simulink model "ScriptDemo"  (R2022b)
settings: configuration reference "TmVcThermal_Configuration_sub" (kept outside this file)
undefined symbols (not defined in the file): aaaa, bbbb, cTmComprCtrl_D_u8HvacFlowTable_db, cTmComprCtrl_D_u8HvacFlowTable_sw, cTmComprCtrl_n_i16ChillCmpIMax, cTmComprCtrl_n_i16ChillCmpIMin, cTmComprCtrl_n_i16ChillCmpIMin666, cTmComprCtrl_n_i16ChillCmpPMax, cTmComprCtrl_n_i16ChillCmpPMin, cTmComprCtrl_n_i16CmpChillCoolRpmKiMax, cTmComprCtrl_n_i16CmpChillCoolRpmKiMin, cTmComprCtrl_n_i16CmpChillCoolRpmKpMax, cTmComprCtrl_n_i16CmpChillCoolRpmKpMin, cTmComprCtrl_n_i16CmpCoolRpmKiMax, cTmComprCtrl_n_i16CmpCoolRpmKiMin, cTmComprCtrl_n_i16CmpCoolRpmKpMax, cTmComprCtrl_n_i16CmpCoolRpmKpMin, cTmComprCtrl_n_i16SM4CmpHeatKiMax, cTmComprCtrl_n_i16SM4CmpHeatKiMin, cTmComprCtrl_n_i16SM4CmpHeatKpMax, cTmComprCtrl_n_i16SM4CmpHeatKpMin, cTmComprCtrl_n_i16SM5CmpHeatKiMax, cTmComprCtrl_n_i16SM5CmpHeatKiMin, cTmComprCtrl_n_i16SM5CmpHeatKpMax, cTmComprCtrl_n_i16SM5CmpHeatKpMin, cTmComprCtrl_n_i16SM6CmpHeatKiMax, cTmComprCtrl_n_i16SM6CmpHeatKiMin, cTmComprCtrl_n_i16SM6CmpHeatKpMax, cTmComprCtrl_n_i16SM6CmpHeatKpMin, cTmComprCtrl_n_u16CmpMaxSpdFanFltLimt, cTmComprCtrl_n_u16CmpMaxSpdLoSidePFltLimt, cTmComprCtrl_n_u16CmpMaxSpdSensorFltLimt, cTmComprCtrl_n_u16CompMinRpm, cTmComprCtrl_n_u16CompRpmIncThres, cTmComprCtrl_t_u16BattCooltFFPeriod, cTmComprCtrl_t_u16BattCooltPIPeriod, cTmComprCtrl_t_u16CmpCoolFFPeriod, cTmComprCtrl_t_u16CmpCoolPIPeriod, cTmComprCtrl_t_u16CoolCmpChillFFPeriod, cTmComprCtrl_t_u16CoolCmpChillPIPeriod, cTmComprCtrl_t_u16SM4CmpHeatFFPeriod, cTmComprCtrl_t_u16SM4CmpHeatPIPeriod, cTmComprCtrl_t_u16SM5CmpHeatFFPeriod, cTmComprCtrl_t_u16SM5CmpHeatPIPeriod, cTmComprCtrl_t_u16SM6CmpHeatFFPeriod, cTmComprCtrl_t_u16SM6CmpHeatPIPeriod, cTmComprCtrl_Te_EvapClearInteg, cTmComprCtrl_Te_i16HpReqTempSaturoffset, cTmComprCtrl_Te_i16SatLpReplaceDiff, cTmComprCtrl_Te_i16SM3BatDiffStartEvapDecOffset, cTmComprCtrl_Te_i16SM3EvapLo, cTmComprCtrl_Te_i16SM3TBatDiffEntEvapDecOffset, cTmComprCtrl_Te_i16SM3TBatDiffEntEvapDecOffsetQuit, cTmComprCtrl_Te_s32ErrCmpChillPIContinueCoolH, cTmComprCtrl_Te_s32ErrCmpChillPIContinueCoolL, cTmComprCtrl_Te_s32ErrCmpPIContinueChillH, cTmComprCtrl_Te_s32ErrCmpPIContinueChillL, cTmComprCtrl_Te_s32ErrCmpPIContinueCoolH, cTmComprCtrl_Te_s32ErrCmpPIContinueCoolL, cTmComprCtrl_Te_s32ErrCmpPIContinueHeatH ... (+398)
libraries: simulink x782, PCMULib x640, simulink_need_slupdate x4
(part 31 of 41)

== system ScriptDemo/Create/createMerge/After/SM2SM22/SM2_Kp/Osa/Subsystem1 ==
  In1 : Inport  OutDataTypeStr=int16
  Abs : Abs  OutDataTypeStr=single  SaturateOnIntegerOverflow=off
  Add6 : Sum  Inputs=+-  OutDataTypeStr=int16
  Compare To Constant : simulink/Logic and Bit Operations/Compare To Constant  relop=>=  const=0  OutDataTypeStr=boolean
  Compare To Constant1 : simulink/Logic and Bit Operations/Compare To Constant  relop=<=  const=10  OutDataTypeStr=boolean
  Constant6 : Constant  Value=0  OutDataTypeStr=uint16
  Constant7 : Constant  Value=10  OutDataTypeStr=uint16
  Logical Operator : Logic  AllPortsSameDT=off  OutDataTypeStr=boolean
  Switch : Switch  Criteria=u2 ~= 0  SaturateOnIntegerOverflow=off  InputSameDT=off
  Out1 : Outport
  wires:
  Add6/1 -> Switch/1
  Logical Operator/1 -> Switch/2
  Constant6/1 -> Switch/3
  Abs/1 -> Add6/2, Compare To Constant/1, Compare To Constant1/1
  Constant7/1 -> Add6/1
  Switch/1 -> Out1/1
  Compare To Constant1/1 -> Logical Operator/2
  Compare To Constant/1 -> Logical Operator/1
  In1/1 -> Abs/1

== system ScriptDemo/Create/createMerge/After/SM2SM22/SM2_Kp/Osa/Subsystem2 ==
  In1 : Inport  OutDataTypeStr=int16
  Abs : Abs  OutDataTypeStr=uint16  SaturateOnIntegerOverflow=off
  Add6 : Sum  Inputs=+-  OutDataTypeStr=int16
  Compare To Constant : simulink/Logic and Bit Operations/Compare To Constant  relop=>=  const=0  OutDataTypeStr=boolean
  Compare To Constant1 : simulink/Logic and Bit Operations/Compare To Constant  relop=<=  const=10  OutDataTypeStr=boolean
  Constant6 : Constant  Value=0  OutDataTypeStr=uint16
  Constant7 : Constant  Value=10  OutDataTypeStr=uint16
  Logical Operator : Logic  AllPortsSameDT=off  OutDataTypeStr=boolean
  Switch : Switch  Criteria=u2 ~= 0  SaturateOnIntegerOverflow=off  InputSameDT=off
  Out1 : Outport
  wires:
  Add6/1 -> Switch/1
  Logical Operator/1 -> Switch/2
  Constant6/1 -> Switch/3
  Abs/1 -> Add6/2, Compare To Constant/1, Compare To Constant1/1
  Constant7/1 -> Add6/1
  Switch/1 -> Out1/1
  Compare To Constant1/1 -> Logical Operator/2
  Compare To Constant/1 -> Logical Operator/1
  In1/1 -> Abs/1

== system ScriptDemo/Create/createMerge/After/SM2SM22/SM2_Kp/Osa/Subsystem3 ==
  In1 : Inport  OutDataTypeStr=int16
  Abs : Abs  OutDataTypeStr=uint16  SaturateOnIntegerOverflow=off
  Add6 : Sum  Inputs=+-  OutDataTypeStr=int16
  Compare To Constant : simulink/Logic and Bit Operations/Compare To Constant  relop=>=  const=0  OutDataTypeStr=boolean
  Compare To Constant1 : simulink/Logic and Bit Operations/Compare To Constant  relop=<=  const=10  OutDataTypeStr=boolean
  Constant6 : Constant  Value=0  OutDataTypeStr=uint16
  Constant7 : Constant  Value=10  OutDataTypeStr=uint16
  Logical Operator : Logic  AllPortsSameDT=off  OutDataTypeStr=boolean
  Switch : Switch  Criteria=u2 ~= 0  SaturateOnIntegerOverflow=off  InputSameDT=off
  Out1 : Outport
  wires:
  Add6/1 -> Switch/1
  Logical Operator/1 -> Switch/2
  Constant6/1 -> Switch/3
  Abs/1 -> Add6/2, Compare To Constant/1, Compare To Constant1/1
  Constant7/1 -> Add6/1
  Switch/1 -> Out1/1
  Compare To Constant1/1 -> Logical Operator/2
  Compare To Constant/1 -> Logical Operator/1
  In1/1 -> Abs/1

== system ScriptDemo/Create/createMerge/After/SM2SM22/SM2_Kp/Osa/Subsystem4 ==
  In1 : Inport  OutDataTypeStr=int16
  Abs : Abs  OutDataTypeStr=uint16  SaturateOnIntegerOverflow=off
  Add6 : Sum  Inputs=+-  OutDataTypeStr=int16
  Compare To Constant : simulink/Logic and Bit Operations/Compare To Constant  relop=>=  const=0  OutDataTypeStr=boolean
  Compare To Constant1 : simulink/Logic and Bit Operations/Compare To Constant  relop=<=  const=10  OutDataTypeStr=boolean
  Constant6 : Constant  Value=0  OutDataTypeStr=uint16
  Constant7 : Constant  Value=10  OutDataTypeStr=uint16
  Logical Operator : Logic  AllPortsSameDT=off  OutDataTypeStr=boolean
  Switch : Switch  Criteria=u2 ~= 0  SaturateOnIntegerOverflow=off  InputSameDT=off
  Out1 : Outport
  wires:
  Add6/1 -> Switch/1
  Logical Operator/1 -> Switch/2
  Constant6/1 -> Switch/3
  Abs/1 -> Add6/2, Compare To Constant/1, Compare To Constant1/1
  Constant7/1 -> Add6/1
  Switch/1 -> Out1/1
  Compare To Constant1/1 -> Logical Operator/2
  Compare To Constant/1 -> Logical Operator/1
  In1/1 -> Abs/1

== system ScriptDemo/Create/createMerge/After/SM2SM22/SM2_Kp/Osa/Subsystem5 ==
  In1 : Inport  OutDataTypeStr=int16
  Abs : Abs  OutDataTypeStr=uint16  SaturateOnIntegerOverflow=off
  Add6 : Sum  Inputs=+-  OutDataTypeStr=int16
  Compare To Constant : simulink/Logic and Bit Operations/Compare To Constant  relop=>=  const=0  OutDataTypeStr=boolean
  Compare To Constant1 : simulink/Logic and Bit Operations/Compare To Constant  relop=<=  const=10  OutDataTypeStr=boolean
  Constant6 : Constant  Value=0  OutDataTypeStr=uint16
  Constant7 : Constant  Value=10  OutDataTypeStr=uint16
  Logical Operator : Logic  AllPortsSameDT=off  OutDataTypeStr=boolean
  Switch : Switch  Criteria=u2 ~= 0  SaturateOnIntegerOverflow=off  InputSameDT=off
  Out1 : Outport
  wires:
  Add6/1 -> Switch/1
  Logical Operator/1 -> Switch/2
  Constant6/1 -> Switch/3
  Abs/1 -> Add6/2, Compare To Constant/1, Compare To Constant1/1
  Constant7/1 -> Add6/1
  Switch/1 -> Out1/1
  Compare To Constant1/1 -> Logical Operator/2
  Compare To Constant/1 -> Logical Operator/1
  In1/1 -> Abs/1

== system ScriptDemo/Create/createMerge/After/SM2SM22/SM2_Kp/Osa/XCP ==
  md_u8Blw : Inport
  Constant1 : Constant  Value=BlwHeatLevel_db
      settings: AttributesFormatString=%<Value>
  Constant28 : Constant  Value=BlwHeatLevel_sw
      settings: AttributesFormatString=%<Value>
  Switch : Switch  Criteria=u2 ~= 0  SaturateOnIntegerOverflow=off  InputSameDT=off
  Out1 : Outport
  wires:
  md_u8Blw/1 -> Switch/3
  Switch/1 -> Out1/1
  Constant28/1 -> Switch/2
  Constant1/1 -> Switch/1

== system ScriptDemo/Create/createMerge/After/SM2SM22/SM2_Kp/Rec/Subsystem1 ==
  In1 : Inport  OutDataTypeStr=int16
  Abs : Abs  OutDataTypeStr=single  SaturateOnIntegerOverflow=off
  Add6 : Sum  Inputs=+-  OutDataTypeStr=int16
  Compare To Constant : simulink/Logic and Bit Operations/Compare To Constant  relop=>=  const=0  OutDataTypeStr=boolean
  Compare To Constant1 : simulink/Logic and Bit Operations/Compare To Constant  relop=<=  const=10  OutDataTypeStr=boolean
  Constant6 : Constant  Value=0  OutDataTypeStr=uint16
  Constant7 : Constant  Value=10  OutDataTypeStr=uint16
  Logical Operator : Logic  AllPortsSameDT=off  OutDataTypeStr=boolean
  Switch : Switch  Criteria=u2 ~= 0  SaturateOnIntegerOverflow=off  InputSameDT=off
  Out1 : Outport
  wires:
  Add6/1 -> Switch/1
  Logical Operator/1 -> Switch/2
  Constant6/1 -> Switch/3
  Abs/1 -> Add6/2, Compare To Constant/1, Compare To Constant1/1
  Constant7/1 -> Add6/1
  Switch/1 -> Out1/1
  Compare To Constant1/1 -> Logical Operator/2
  Compare To Constant/1 -> Logical Operator/1
  In1/1 -> Abs/1

== system ScriptDemo/Create/createMerge/After/SM2SM22/SM2_Kp/Rec/Subsystem2 ==
  In1 : Inport  OutDataTypeStr=int16
  Abs : Abs  OutDataTypeStr=uint16  SaturateOnIntegerOverflow=off
  Add6 : Sum  Inputs=+-  OutDataTypeStr=int16
  Compare To Constant : simulink/Logic and Bit Operations/Compare To Constant  relop=>=  const=0  OutDataTypeStr=boolean
  Compare To Constant1 : simulink/Logic and Bit Operations/Compare To Constant  relop=<=  const=10  OutDataTypeStr=boolean
  Constant6 : Constant  Value=0  OutDataTypeStr=uint16
  Constant7 : Constant  Value=10  OutDataTypeStr=uint16
  Logical Operator : Logic  AllPortsSameDT=off  OutDataTypeStr=boolean
  Switch : Switch  Criteria=u2 ~= 0  SaturateOnIntegerOverflow=off  InputSameDT=off
  Out1 : Outport
  wires:
  Add6/1 -> Switch/1
  Logical Operator/1 -> Switch/2
  Constant6/1 -> Switch/3
  Abs/1 -> Add6/2, Compare To Constant/1, Compare To Constant1/1
  Constant7/1 -> Add6/1
  Switch/1 -> Out1/1
  Compare To Constant1/1 -> Logical Operator/2
  Compare To Constant/1 -> Logical Operator/1
  In1/1 -> Abs/1

== system ScriptDemo/Create/createMerge/After/SM2SM22/SM2_Kp/Rec/Subsystem3 ==
  In1 : Inport  OutDataTypeStr=int16
  Abs : Abs  OutDataTypeStr=uint16  SaturateOnIntegerOverflow=off
  Add6 : Sum  Inputs=+-  OutDataTypeStr=int16
  Compare To Constant : simulink/Logic and Bit Operations/Compare To Constant  relop=>=  const=0  OutDataTypeStr=boolean
  Compare To Constant1 : simulink/Logic and Bit Operations/Compare To Constant  relop=<=  const=10  OutDataTypeStr=boolean
  Constant6 : Constant  Value=0  OutDataTypeStr=uint16
  Constant7 : Constant  Value=10  OutDataTypeStr=uint16
  Logical Operator : Logic  AllPortsSameDT=off  OutDataTypeStr=boolean
  Switch : Switch  Criteria=u2 ~= 0  SaturateOnIntegerOverflow=off  InputSameDT=off
  Out1 : Outport
  wires:
  Add6/1 -> Switch/1
  Logical Operator/1 -> Switch/2
  Constant6/1 -> Switch/3
  Abs/1 -> Add6/2, Compare To Constant/1, Compare To Constant1/1
  Constant7/1 -> Add6/1
  Switch/1 -> Out1/1
  Compare To Constant1/1 -> Logical Operator/2
  Compare To Constant/1 -> Logical Operator/1
  In1/1 -> Abs/1

== system ScriptDemo/Create/createMerge/After/SM2SM22/SM2_Kp/Rec/Subsystem4 ==
  In1 : Inport  OutDataTypeStr=int16
  Abs : Abs  OutDataTypeStr=uint16  SaturateOnIntegerOverflow=off
  Add6 : Sum  Inputs=+-  OutDataTypeStr=int16
  Compare To Constant : simulink/Logic and Bit Operations/Compare To Constant  relop=>=  const=0  OutDataTypeStr=boolean
  Compare To Constant1 : simulink/Logic and Bit Operations/Compare To Constant  relop=<=  const=10  OutDataTypeStr=boolean
  Constant6 : Constant  Value=0  OutDataTypeStr=uint16
  Constant7 : Constant  Value=10  OutDataTypeStr=uint16
  Logical Operator : Logic  AllPortsSameDT=off  OutDataTypeStr=boolean
  Switch : Switch  Criteria=u2 ~= 0  SaturateOnIntegerOverflow=off  InputSameDT=off
  Out1 : Outport
  wires:
  Add6/1 -> Switch/1
  Logical Operator/1 -> Switch/2
  Constant6/1 -> Switch/3
  Abs/1 -> Add6/2, Compare To Constant/1, Compare To Constant1/1
  Constant7/1 -> Add6/1
  Switch/1 -> Out1/1
  Compare To Constant1/1 -> Logical Operator/2
  Compare To Constant/1 -> Logical Operator/1
  In1/1 -> Abs/1

== system ScriptDemo/Create/createMerge/After/SM2SM22/SM2_Kp/Rec/Subsystem5 ==
  In1 : Inport  OutDataTypeStr=int16
  Abs : Abs  OutDataTypeStr=uint16  SaturateOnIntegerOverflow=off
  Add6 : Sum  Inputs=+-  OutDataTypeStr=int16
  Compare To Constant : simulink/Logic and Bit Operations/Compare To Constant  relop=>=  const=0  OutDataTypeStr=boolean
  Compare To Constant1 : simulink/Logic and Bit Operations/Compare To Constant  relop=<=  const=10  OutDataTypeStr=boolean
  Constant6 : Constant  Value=0  OutDataTypeStr=uint16
  Constant7 : Constant  Value=10  OutDataTypeStr=uint16
  Logical Operator : Logic  AllPortsSameDT=off  OutDataTypeStr=boolean
  Switch : Switch  Criteria=u2 ~= 0  SaturateOnIntegerOverflow=off  InputSameDT=off
  Out1 : Outport
  wires:
  Add6/1 -> Switch/1
  Logical Operator/1 -> Switch/2
  Constant6/1 -> Switch/3
  Abs/1 -> Add6/2, Compare To Constant/1, Compare To Constant1/1
  Constant7/1 -> Add6/1
  Switch/1 -> Out1/1
  Compare To Constant1/1 -> Logical Operator/2
  Compare To Constant/1 -> Logical Operator/1
  In1/1 -> Abs/1

== system ScriptDemo/Create/createMerge/After/SM2SM22/SM2_Kp/Rec/XCP ==
  md_u8Blw : Inport
  Constant1 : Constant  Value=BlwHeatLevel_db
      settings: AttributesFormatString=%<Value>
  Constant28 : Constant  Value=BlwHeatLevel_sw
      settings: AttributesFormatString=%<Value>
  Switch : Switch  Criteria=u2 ~= 0  SaturateOnIntegerOverflow=off  InputSameDT=off
  Out1 : Outport
  wires:
  md_u8Blw/1 -> Switch/3
  Switch/1 -> Out1/1
  Constant28/1 -> Switch/2
  Constant1/1 -> Switch/1

== system ScriptDemo/Create/createMerge/After/SM3SM23/ID26262_SM3FF/SM1FFEnable/BevvFFPeriod ==
  Counter_Reset : Inport
  Add : Sum
  Add1 : Sum  Inputs=+-
  Constant : Constant  Value=CounterLim
  Constant1 : Constant  Value=cTmSwArch_t_s32SampleTime
      settings: AttributesFormatString=%<Value>
  Constant2 : Constant  Value=0  OutDataTypeStr=single
  Constant50 : Constant  Value=cTmSwArch_t_s32SampleTime
      settings: AttributesFormatString=%<Value>
  Logical Operator : Logic  Operator=OR  AllPortsSameDT=off  OutDataTypeStr=boolean
  Relational Operator : RelationalOperator  OutDataTypeStr=boolean  RndMeth=Simplest  InputSameDT=off
  Switch : Switch  Criteria=u2 ~= 0  SaturateOnIntegerOverflow=off  InputSameDT=off
  Switch1 : Switch  Criteria=u2 ~= 0  SaturateOnIntegerOverflow=off  InputSameDT=off
  Unit Delay : UnitDelay  SampleTime=-1  HasFrameUpgradeWarning=on
  Unit Delay1 : UnitDelay  SampleTime=-1  HasFrameUpgradeWarning=on
  Counter_Trig : Outport
  wires:
  Relational Operator/1 -> Unit Delay1/1, Counter_Trig/1
  [CounterLim] -> Relational Operator/2
  Add/1 -> Unit Delay/1, Relational Operator/1
  Unit Delay/1 -> Switch/3
  Switch/1 -> Add/2
  Constant1/1 -> Add/1
  Logical Operator/1 -> Switch/2
  Counter_Reset/1 -> Switch1/2, Logical Operator/1
  Unit Delay1/1 -> Logical Operator/2
  Constant2/1 -> Switch1/3
  Switch1/1 -> Switch/1
  Add1/1 -> Switch1/1
  Constant50/1 -> Add1/2
  Constant/1 -> [CounterLim]
  [CounterLim] -> Add1/1

== system ScriptDemo/Create/createMerge/After/SM3SM23/ID26262_SM3FF/SM2FFEnable/PeriodTrig ==
  Counter_Reset : Inport
  Add : Sum
  Add1 : Sum  Inputs=+-
  Constant : Constant  Value=CounterLim
  Constant1 : Constant  Value=cTmSwArch_t_s32SampleTime
      settings: AttributesFormatString=%<Value>
  Constant2 : Constant  Value=0  OutDataTypeStr=single
  Constant50 : Constant  Value=cTmSwArch_t_s32SampleTime
      settings: AttributesFormatString=%<Value>
  Logical Operator : Logic  Operator=OR  AllPortsSameDT=off  OutDataTypeStr=boolean
  Relational Operator : RelationalOperator  OutDataTypeStr=boolean  RndMeth=Simplest  InputSameDT=off
  Switch : Switch  Criteria=u2 ~= 0  SaturateOnIntegerOverflow=off  InputSameDT=off
  Switch1 : Switch  Criteria=u2 ~= 0  SaturateOnIntegerOverflow=off  InputSameDT=off
  Unit Delay : UnitDelay  SampleTime=-1  HasFrameUpgradeWarning=on
  Unit Delay1 : UnitDelay  SampleTime=-1  HasFrameUpgradeWarning=on
  Counter_Trig : Outport
  wires:
  Relational Operator/1 -> Unit Delay1/1, Counter_Trig/1
  [CounterLim] -> Relational Operator/2
  Add/1 -> Unit Delay/1, Relational Operator/1
  Unit Delay/1 -> Switch/3
  Switch/1 -> Add/2
  Constant1/1 -> Add/1
  Logical Operator/1 -> Switch/2
  Counter_Reset/1 -> Switch1/2, Logical Operator/1
  Unit Delay1/1 -> Logical Operator/2
  Constant2/1 -> Switch1/3
  Switch1/1 -> Switch/1
  Add1/1 -> Switch1/1
  Constant50/1 -> Add1/2
  Constant/1 -> [CounterLim]
  [CounterLim] -> Add1/1

== system ScriptDemo/Create/createMerge/After/SM3SM23/ID26262_SM3FF/SM3SM2FF/Flow2RpmOsa ==
  md_u8Blw : Inport
  breakpoint1 : Inport  Port=2
  breakpoint2 : Inport  Port=3
  2-D Lookup Table5 : Lookup_n-D  BreakpointsForDimension1=FFBlw1_Y  BreakpointsForDimension2=FFBlw1_X  BreakpointsForDimension1DataTypeStr=Inherit: Inherit from 'Breakpoint data'  BreakpointsForDimension2DataTypeStr=Inherit: Inherit from 'Breakpoint data'  Table=FFBlw1  TableDataTypeStr=Inherit: Inherit from 'Table data'  ExtrapMethod=Clip  InternalRulePriority=Speed  OutDataTypeStr=Inherit: Inherit from 'Table data'  RndMeth=Simplest
      settings: InputPortMap=u0,u1
  2-D Lookup Table6 : Lookup_n-D  BreakpointsForDimension1=FFBlw3_Y  BreakpointsForDimension2=FFBlw3_X  BreakpointsForDimension1DataTypeStr=Inherit: Inherit from 'Breakpoint data'  BreakpointsForDimension2DataTypeStr=Inherit: Inherit from 'Breakpoint data'  Table=FFBlw3  TableDataTypeStr=Inherit: Inherit from 'Table data'  ExtrapMethod=Clip  InternalRulePriority=Speed  OutDataTypeStr=Inherit: Inherit from 'Table data'  RndMeth=Simplest
      settings: InputPortMap=u0,u1
  2-D Lookup Table7 : Lookup_n-D  BreakpointsForDimension1=FFBlw5_Y  BreakpointsForDimension2=FFBlw5_X  BreakpointsForDimension1DataTypeStr=Inherit: Inherit from 'Breakpoint data'  BreakpointsForDimension2DataTypeStr=Inherit: Inherit from 'Breakpoint data'  Table=FFBlw5  TableDataTypeStr=Inherit: Inherit from 'Table data'  ExtrapMethod=Clip  InternalRulePriority=Speed  OutDataTypeStr=Inherit: Inherit from 'Table data'  RndMeth=Simplest
      settings: InputPortMap=u0,u1
  2-D Lookup Table8 : Lookup_n-D  BreakpointsForDimension1=FFBlw7_Y  BreakpointsForDimension2=FFBlw7_X  BreakpointsForDimension1DataTypeStr=Inherit: Inherit from 'Breakpoint data'  BreakpointsForDimension2DataTypeStr=Inherit: Inherit from 'Breakpoint data'  Table=FFBlw7  TableDataTypeStr=Inherit: Inherit from 'Table data'  ExtrapMethod=Clip  InternalRulePriority=Speed  OutDataTypeStr=Inherit: Inherit from 'Table data'  RndMeth=Simplest
      settings: InputPortMap=u0,u1
  2-D Lookup Table9 : Lookup_n-D  BreakpointsForDimension1=FFBlw9_Y  BreakpointsForDimension2=FFBlw9_X  BreakpointsForDimension1DataTypeStr=Inherit: Inherit from 'Breakpoint data'  BreakpointsForDimension2DataTypeStr=Inherit: Inherit from 'Breakpoint data'  Table=FFBlw9  TableDataTypeStr=Inherit: Inherit from 'Table data'  ExtrapMethod=Clip  InternalRulePriority=Speed  OutDataTypeStr=Inherit: Inherit from 'Table data'  RndMeth=Simplest
      settings: InputPortMap=u0,u1
  Add{2..6} (5 alike) : Sum  Inputs=+-  OutDataTypeStr=int16
  Add7 : Sum  Inputs=+++++
  Constant{,1..4} (5 alike) : Constant  Value=0.1  OutDataTypeStr=single
  Constant5 : Constant  Value=10  OutDataTypeStr=int16
  Constant6 : Constant  Value=20  OutDataTypeStr=int16
  Constant7 : Constant  Value=30  OutDataTypeStr=int16
  Constant8 : Constant  Value=40  OutDataTypeStr=int16
  Constant9 : Constant  Value=50  OutDataTypeStr=int16
  Data Type Conversion : DataTypeConversion  OutDataTypeStr=uint16  SaturateOnIntegerOverflow=off  RndMeth=Floor
  Data Type Conversion1 : DataTypeConversion  OutDataTypeStr=int16  SaturateOnIntegerOverflow=off  RndMeth=Floor
  Product{,1..9} (10 alike) : Product  OutDataTypeStr=single
  Subsystem1 : Subsystem
  Subsystem2 : Subsystem
  Subsystem3 : Subsystem
  Subsystem4 : Subsystem
  Subsystem5 : Subsystem
  XCP : Subsystem
  Flow2Rpm : Outport
  wires:
  Subsystem1/1(Out1) -> Product/2
  Product2/1 -> Product7/2
  [breakpoint2] -> 2-D Lookup Table5/2
  Product4/1 -> Product9/2
  Product9/1 -> Add7/5
  [breakpoint1] -> 2-D Lookup Table7/1
  Constant9/1 -> Add6/1
  [breakpoint1] -> 2-D Lookup Table9/1
  [breakpoint1] -> 2-D Lookup Table5/1
  [breakpoint1] -> 2-D Lookup Table6/1
  Product5/1 -> Add7/1
  2-D Lookup Table7/1 -> Product2/1
  Data Type Conversion1/1 -> Add4/2, Add6/2, Add5/2, Add3/2, Add2/2
  [breakpoint2] -> 2-D Lookup Table8/2
  Product/1 -> Product5/2
  Subsystem5/1(Out1) -> Product4/2
  [breakpoint2] -> 2-D Lookup Table7/2
  Subsystem2/1(Out1) -> Product1/2
  Constant8/1 -> Add5/1
  Product8/1 -> Add7/4
  Constant7/1 -> Add4/1
  Add4/1 -> Subsystem3/1(In1)
  Subsystem3/1(Out1) -> Product2/2
  Subsystem4/1(Out1) -> Product3/2
  Product1/1 -> Product6/2
  Add2/1 -> Subsystem1/1(In1)
  [breakpoint1] -> 2-D Lookup Table8/1
  [breakpoint2] -> 2-D Lookup Table6/2
  2-D Lookup Table5/1 -> Product/1
  Constant5/1 -> Add2/1
  2-D Lookup Table8/1 -> Product3/1
  Constant6/1 -> Add3/1
  Add6/1 -> Subsystem5/1(In1)
  Add5/1 -> Subsystem4/1(In1)
  Product3/1 -> Product8/2
  [breakpoint2] -> 2-D Lookup Table9/2
  Add3/1 -> Subsystem2/1(In1)
  Add7/1 -> Data Type Conversion/1
  2-D Lookup Table6/1 -> Product1/1
  Product7/1 -> Add7/3
  2-D Lookup Table9/1 -> Product4/1
  Product6/1 -> Add7/2
  breakpoint1/1 -> [breakpoint1]
  breakpoint2/1 -> [breakpoint2]
  XCP/1(Out1) -> Data Type Conversion1/1
  Constant/1 -> Product5/1
  Constant1/1 -> Product6/1
  Constant2/1 -> Product7/1
  Constant3/1 -> Product8/1
  Constant4/1 -> Product9/1
  md_u8Blw/1 -> XCP/1(md_u8Blw)
  Data Type Conversion/1 -> Flow2Rpm/1

== system ScriptDemo/Create/createMerge/After/SM3SM23/ID26262_SM3FF/SM3SM2FF/Flow2RpmOsa1 ==
  md_u8Blw : Inport
  breakpoint1 : Inport  Port=2
  breakpoint2 : Inport  Port=3
  2-D Lookup Table5 : Lookup_n-D  BreakpointsForDimension1=FFBlw1_Y  BreakpointsForDimension2=FFBlw1_X  BreakpointsForDimension1DataTypeStr=Inherit: Inherit from 'Breakpoint data'  BreakpointsForDimension2DataTypeStr=Inherit: Inherit from 'Breakpoint data'  Table=FFBlw1  TableDataTypeStr=Inherit: Inherit from 'Table data'  ExtrapMethod=Clip  InternalRulePriority=Speed  OutDataTypeStr=Inherit: Inherit from 'Table data'  RndMeth=Simplest
      settings: InputPortMap=u0,u1
  2-D Lookup Table6 : Lookup_n-D  BreakpointsForDimension1=FFBlw3_Y  BreakpointsForDimension2=FFBlw3_X  BreakpointsForDimension1DataTypeStr=Inherit: Inherit from 'Breakpoint data'  BreakpointsForDimension2DataTypeStr=Inherit: Inherit from 'Breakpoint data'  Table=FFBlw3  TableDataTypeStr=Inherit: Inherit from 'Table data'  ExtrapMethod=Clip  InternalRulePriority=Speed  OutDataTypeStr=Inherit: Inherit from 'Table data'  RndMeth=Simplest
      settings: InputPortMap=u0,u1
  2-D Lookup Table7 : Lookup_n-D  BreakpointsForDimension1=FFBlw5_Y  BreakpointsForDimension2=FFBlw5_X  BreakpointsForDimension1DataTypeStr=Inherit: Inherit from 'Breakpoint data'  BreakpointsForDimension2DataTypeStr=Inherit: Inherit from 'Breakpoint data'  Table=FFBlw5  TableDataTypeStr=Inherit: Inherit from 'Table data'  ExtrapMethod=Clip  InternalRulePriority=Speed  OutDataTypeStr=Inherit: Inherit from 'Table data'  RndMeth=Simplest
      settings: InputPortMap=u0,u1
  2-D Lookup Table8 : Lookup_n-D  BreakpointsForDimension1=FFBlw7_Y  BreakpointsForDimension2=FFBlw7_X  BreakpointsForDimension1DataTypeStr=Inherit: Inherit from 'Breakpoint data'  BreakpointsForDimension2DataTypeStr=Inherit: Inherit from 'Breakpoint data'  Table=FFBlw7  TableDataTypeStr=Inherit: Inherit from 'Table data'  ExtrapMethod=Clip  InternalRulePriority=Speed  OutDataTypeStr=Inherit: Inherit from 'Table data'  RndMeth=Simplest
      settings: InputPortMap=u0,u1
  2-D Lookup Table9 : Lookup_n-D  BreakpointsForDimension1=FFBlw9_Y  BreakpointsForDimension2=FFBlw9_X  BreakpointsForDimension1DataTypeStr=Inherit: Inherit from 'Breakpoint data'  BreakpointsForDimension2DataTypeStr=Inherit: Inherit from 'Breakpoint data'  Table=FFBlw9  TableDataTypeStr=Inherit: Inherit from 'Table data'  ExtrapMethod=Clip  InternalRulePriority=Speed  OutDataTypeStr=Inherit: Inherit from 'Table data'  RndMeth=Simplest
      settings: InputPortMap=u0,u1
  Add{2..6} (5 alike) : Sum  Inputs=+-  OutDataTypeStr=int16
  Add7 : Sum  Inputs=+++++
  Constant{,1..4} (5 alike) : Constant  Value=0.1  OutDataTypeStr=single
  Constant5 : Constant  Value=10  OutDataTypeStr=int16
  Constant6 : Constant  Value=20  OutDataTypeStr=int16
  Constant7 : Constant  Value=30  OutDataTypeStr=int16
  Constant8 : Constant  Value=40  OutDataTypeStr=int16
  Constant9 : Constant  Value=50  OutDataTypeStr=int16
  Data Type Conversion : DataTypeConversion  OutDataTypeStr=uint16  SaturateOnIntegerOverflow=off  RndMeth=Floor
  Data Type Conversion1 : DataTypeConversion  OutDataTypeStr=int16  SaturateOnIntegerOverflow=off  RndMeth=Floor
  Product{,1..9} (10 alike) : Product  OutDataTypeStr=single
  Subsystem1 : Subsystem
  Subsystem2 : Subsystem
  Subsystem3 : Subsystem
  Subsystem4 : Subsystem
  Subsystem5 : Subsystem
  XCP : Subsystem
  Flow2Rpm : Outport
  wires:
  Subsystem1/1(Out1) -> Product/2
  Product2/1 -> Product7/2
  [breakpoint2] -> 2-D Lookup Table5/2
  Product4/1 -> Product9/2
  Product9/1 -> Add7/5
  [breakpoint1] -> 2-D Lookup Table7/1
  Constant9/1 -> Add6/1
  [breakpoint1] -> 2-D Lookup Table9/1
  [breakpoint1] -> 2-D Lookup Table5/1
  [breakpoint1] -> 2-D Lookup Table6/1
  Product5/1 -> Add7/1
  2-D Lookup Table7/1 -> Product2/1
  Data Type Conversion1/1 -> Add4/2, Add6/2, Add5/2, Add3/2, Add2/2
  [breakpoint2] -> 2-D Lookup Table8/2
  Product/1 -> Product5/2
  Subsystem5/1(Out1) -> Product4/2
  [breakpoint2] -> 2-D Lookup Table7/2
  Subsystem2/1(Out1) -> Product1/2
  Constant8/1 -> Add5/1
  Product8/1 -> Add7/4
  Constant7/1 -> Add4/1
  Add4/1 -> Subsystem3/1(In1)
  Subsystem3/1(Out1) -> Product2/2
  Subsystem4/1(Out1) -> Product3/2
  Product1/1 -> Product6/2
  Add2/1 -> Subsystem1/1(In1)
  [breakpoint1] -> 2-D Lookup Table8/1
  [breakpoint2] -> 2-D Lookup Table6/2
  2-D Lookup Table5/1 -> Product/1
  Constant5/1 -> Add2/1
  2-D Lookup Table8/1 -> Product3/1
  Constant6/1 -> Add3/1
  Add6/1 -> Subsystem5/1(In1)
  Add5/1 -> Subsystem4/1(In1)
  Product3/1 -> Product8/2
  [breakpoint2] -> 2-D Lookup Table9/2
  Add3/1 -> Subsystem2/1(In1)
  Add7/1 -> Data Type Conversion/1
  2-D Lookup Table6/1 -> Product1/1
  Product7/1 -> Add7/3
  2-D Lookup Table9/1 -> Product4/1
  Product6/1 -> Add7/2
  breakpoint1/1 -> [breakpoint1]
  breakpoint2/1 -> [breakpoint2]
  XCP/1(Out1) -> Data Type Conversion1/1
  Constant/1 -> Product5/1
  Constant1/1 -> Product6/1
  Constant2/1 -> Product7/1
  Constant3/1 -> Product8/1
  Constant4/1 -> Product9/1
  md_u8Blw/1 -> XCP/1(md_u8Blw)
  Data Type Conversion/1 -> Flow2Rpm/1

== system ScriptDemo/Create/createMerge/After/SM3SM23/ID26262_SM3FF/SM3SM2FF/Flow2RpmRec ==
  md_u8Blw : Inport
  breakpoint1 : Inport  Port=2
  breakpoint2 : Inport  Port=3
  2-D Lookup Table5 : Lookup_n-D  BreakpointsForDimension1=FFBlw1_Y  BreakpointsForDimension2=FFBlw1_X  BreakpointsForDimension1DataTypeStr=Inherit: Inherit from 'Breakpoint data'  BreakpointsForDimension2DataTypeStr=Inherit: Inherit from 'Breakpoint data'  Table=FFBlw1  TableDataTypeStr=Inherit: Inherit from 'Table data'  ExtrapMethod=Clip  InternalRulePriority=Speed  OutDataTypeStr=Inherit: Inherit from 'Table data'  RndMeth=Simplest
      settings: InputPortMap=u0,u1
  2-D Lookup Table6 : Lookup_n-D  BreakpointsForDimension1=FFBlw3_Y  BreakpointsForDimension2=FFBlw3_X  BreakpointsForDimension1DataTypeStr=Inherit: Inherit from 'Breakpoint data'  BreakpointsForDimension2DataTypeStr=Inherit: Inherit from 'Breakpoint data'  Table=FFBlw3  TableDataTypeStr=Inherit: Inherit from 'Table data'  ExtrapMethod=Clip  InternalRulePriority=Speed  OutDataTypeStr=Inherit: Inherit from 'Table data'  RndMeth=Simplest
      settings: InputPortMap=u0,u1
  2-D Lookup Table7 : Lookup_n-D  BreakpointsForDimension1=FFBlw5_Y  BreakpointsForDimension2=FFBlw5_X  BreakpointsForDimension1DataTypeStr=Inherit: Inherit from 'Breakpoint data'  BreakpointsForDimension2DataTypeStr=Inherit: Inherit from 'Breakpoint data'  Table=FFBlw5  TableDataTypeStr=Inherit: Inherit from 'Table data'  ExtrapMethod=Clip  InternalRulePriority=Speed  OutDataTypeStr=Inherit: Inherit from 'Table data'  RndMeth=Simplest
      settings: InputPortMap=u0,u1
  2-D Lookup Table8 : Lookup_n-D  BreakpointsForDimension1=FFBlw7_Y  BreakpointsForDimension2=FFBlw7_X  BreakpointsForDimension1DataTypeStr=Inherit: Inherit from 'Breakpoint data'  BreakpointsForDimension2DataTypeStr=Inherit: Inherit from 'Breakpoint data'  Table=FFBlw7  TableDataTypeStr=Inherit: Inherit from 'Table data'  ExtrapMethod=Clip  InternalRulePriority=Speed  OutDataTypeStr=Inherit: Inherit from 'Table data'  RndMeth=Simplest
      settings: InputPortMap=u0,u1
  2-D Lookup Table9 : Lookup_n-D  BreakpointsForDimension1=FFBlw9_Y  BreakpointsForDimension2=FFBlw9_X  BreakpointsForDimension1DataTypeStr=Inherit: Inherit from 'Breakpoint data'  BreakpointsForDimension2DataTypeStr=Inherit: Inherit from 'Breakpoint data'  Table=FFBlw9  TableDataTypeStr=Inherit: Inherit from 'Table data'  ExtrapMethod=Clip  InternalRulePriority=Speed  OutDataTypeStr=Inherit: Inherit from 'Table data'  RndMeth=Simplest
      settings: InputPortMap=u0,u1
  Add{2..6} (5 alike) : Sum  Inputs=+-  OutDataTypeStr=int16
  Add7 : Sum  Inputs=+++++
  Constant{,1..4} (5 alike) : Constant  Value=0.1  OutDataTypeStr=single
  Constant5 : Constant  Value=10  OutDataTypeStr=int16
  Constant6 : Constant  Value=20  OutDataTypeStr=int16
  Constant7 : Constant  Value=30  OutDataTypeStr=int16
  Constant8 : Constant  Value=40  OutDataTypeStr=int16
  Constant9 : Constant  Value=50  OutDataTypeStr=int16
  Data Type Conversion : DataTypeConversion  OutDataTypeStr=uint16  SaturateOnIntegerOverflow=off  RndMeth=Floor
  Data Type Conversion1 : DataTypeConversion  OutDataTypeStr=int16  SaturateOnIntegerOverflow=off  RndMeth=Floor
  Product{,1..9} (10 alike) : Product  OutDataTypeStr=single
  Subsystem1 : Subsystem
  Subsystem2 : Subsystem
  Subsystem3 : Subsystem
  Subsystem4 : Subsystem
  Subsystem5 : Subsystem
  XCP : Subsystem
  Flow2Rpm : Outport
  wires:
  Subsystem1/1(Out1) -> Product/2
  Product2/1 -> Product7/2
  [breakpoint2] -> 2-D Lookup Table5/2
  Product4/1 -> Product9/2
  Product9/1 -> Add7/5
  [breakpoint1] -> 2-D Lookup Table7/1
  Constant9/1 -> Add6/1
  [breakpoint1] -> 2-D Lookup Table9/1
  [breakpoint1] -> 2-D Lookup Table5/1
  [breakpoint1] -> 2-D Lookup Table6/1
  Product5/1 -> Add7/1
  2-D Lookup Table7/1 -> Product2/1
  Data Type Conversion1/1 -> Add4/2, Add6/2, Add5/2, Add3/2, Add2/2
  [breakpoint2] -> 2-D Lookup Table8/2
  Product/1 -> Product5/2
  Subsystem5/1(Out1) -> Product4/2
  [breakpoint2] -> 2-D Lookup Table7/2
  Subsystem2/1(Out1) -> Product1/2
  Constant8/1 -> Add5/1
  Product8/1 -> Add7/4
  Constant7/1 -> Add4/1
  Add4/1 -> Subsystem3/1(In1)
  Subsystem3/1(Out1) -> Product2/2
  Subsystem4/1(Out1) -> Product3/2
  Product1/1 -> Product6/2
  Add2/1 -> Subsystem1/1(In1)
  [breakpoint1] -> 2-D Lookup Table8/1
  [breakpoint2] -> 2-D Lookup Table6/2
  2-D Lookup Table5/1 -> Product/1
  Constant5/1 -> Add2/1
  2-D Lookup Table8/1 -> Product3/1
  Constant6/1 -> Add3/1
  Add6/1 -> Subsystem5/1(In1)
  Add5/1 -> Subsystem4/1(In1)
  Product3/1 -> Product8/2
  [breakpoint2] -> 2-D Lookup Table9/2
  Add3/1 -> Subsystem2/1(In1)
  Add7/1 -> Data Type Conversion/1
  2-D Lookup Table6/1 -> Product1/1
  Product7/1 -> Add7/3
  2-D Lookup Table9/1 -> Product4/1
  Product6/1 -> Add7/2
  breakpoint1/1 -> [breakpoint1]
  breakpoint2/1 -> [breakpoint2]
  XCP/1(Out1) -> Data Type Conversion1/1
  Constant/1 -> Product5/1
  Constant1/1 -> Product6/1
  Constant2/1 -> Product7/1
  Constant3/1 -> Product8/1
  Constant4/1 -> Product9/1
  md_u8Blw/1 -> XCP/1(md_u8Blw)
  Data Type Conversion/1 -> Flow2Rpm/1

== system ScriptDemo/Create/createMerge/After/SM3SM23/ID26262_SM3FF/SM3SM2FF/Flow2RpmRec1 ==
  md_u8Blw : Inport
  breakpoint1 : Inport  Port=2
  breakpoint2 : Inport  Port=3
  2-D Lookup Table5 : Lookup_n-D  BreakpointsForDimension1=FFBlw1_Y  BreakpointsForDimension2=FFBlw1_X  BreakpointsForDimension1DataTypeStr=Inherit: Inherit from 'Breakpoint data'  BreakpointsForDimension2DataTypeStr=Inherit: Inherit from 'Breakpoint data'  Table=FFBlw1  TableDataTypeStr=Inherit: Inherit from 'Table data'  ExtrapMethod=Clip  InternalRulePriority=Speed  OutDataTypeStr=Inherit: Inherit from 'Table data'  RndMeth=Simplest
      settings: InputPortMap=u0,u1
  2-D Lookup Table6 : Lookup_n-D  BreakpointsForDimension1=FFBlw3_Y  BreakpointsForDimension2=FFBlw3_X  BreakpointsForDimension1DataTypeStr=Inherit: Inherit from 'Breakpoint data'  BreakpointsForDimension2DataTypeStr=Inherit: Inherit from 'Breakpoint data'  Table=FFBlw3  TableDataTypeStr=Inherit: Inherit from 'Table data'  ExtrapMethod=Clip  InternalRulePriority=Speed  OutDataTypeStr=Inherit: Inherit from 'Table data'  RndMeth=Simplest
      settings: InputPortMap=u0,u1
  2-D Lookup Table7 : Lookup_n-D  BreakpointsForDimension1=FFBlw5_Y  BreakpointsForDimension2=FFBlw5_X  BreakpointsForDimension1DataTypeStr=Inherit: Inherit from 'Breakpoint data'  BreakpointsForDimension2DataTypeStr=Inherit: Inherit from 'Breakpoint data'  Table=FFBlw5  TableDataTypeStr=Inherit: Inherit from 'Table data'  ExtrapMethod=Clip  InternalRulePriority=Speed  OutDataTypeStr=Inherit: Inherit from 'Table data'  RndMeth=Simplest
      settings: InputPortMap=u0,u1
  2-D Lookup Table8 : Lookup_n-D  BreakpointsForDimension1=FFBlw7_Y  BreakpointsForDimension2=FFBlw7_X  BreakpointsForDimension1DataTypeStr=Inherit: Inherit from 'Breakpoint data'  BreakpointsForDimension2DataTypeStr=Inherit: Inherit from 'Breakpoint data'  Table=FFBlw7  TableDataTypeStr=Inherit: Inherit from 'Table data'  ExtrapMethod=Clip  InternalRulePriority=Speed  OutDataTypeStr=Inherit: Inherit from 'Table data'  RndMeth=Simplest
      settings: InputPortMap=u0,u1
  2-D Lookup Table9 : Lookup_n-D  BreakpointsForDimension1=FFBlw9_Y  BreakpointsForDimension2=FFBlw9_X  BreakpointsForDimension1DataTypeStr=Inherit: Inherit from 'Breakpoint data'  BreakpointsForDimension2DataTypeStr=Inherit: Inherit from 'Breakpoint data'  Table=FFBlw9  TableDataTypeStr=Inherit: Inherit from 'Table data'  ExtrapMethod=Clip  InternalRulePriority=Speed  OutDataTypeStr=Inherit: Inherit from 'Table data'  RndMeth=Simplest
      settings: InputPortMap=u0,u1
  Add{2..6} (5 alike) : Sum  Inputs=+-  OutDataTypeStr=int16
  Add7 : Sum  Inputs=+++++
  Constant{,1..4} (5 alike) : Constant  Value=0.1  OutDataTypeStr=single
  Constant5 : Constant  Value=10  OutDataTypeStr=int16
  Constant6 : Constant  Value=20  OutDataTypeStr=int16
  Constant7 : Constant  Value=30  OutDataTypeStr=int16
  Constant8 : Constant  Value=40  OutDataTypeStr=int16
  Constant9 : Constant  Value=50  OutDataTypeStr=int16
  Data Type Conversion : DataTypeConversion  OutDataTypeStr=uint16  SaturateOnIntegerOverflow=off  RndMeth=Floor
  Data Type Conversion1 : DataTypeConversion  OutDataTypeStr=int16  SaturateOnIntegerOverflow=off  RndMeth=Floor
  Product{,1..9} (10 alike) : Product  OutDataTypeStr=single
  Subsystem1 : Subsystem
  Subsystem2 : Subsystem
  Subsystem3 : Subsystem
  Subsystem4 : Subsystem
  Subsystem5 : Subsystem
  XCP : Subsystem
  Flow2Rpm : Outport
  wires:
  Subsystem1/1(Out1) -> Product/2
  Product2/1 -> Product7/2
  [breakpoint2] -> 2-D Lookup Table5/2
  Product4/1 -> Product9/2
  Product9/1 -> Add7/5
  [breakpoint1] -> 2-D Lookup Table7/1
  Constant9/1 -> Add6/1
  [breakpoint1] -> 2-D Lookup Table9/1
  [breakpoint1] -> 2-D Lookup Table5/1
  [breakpoint1] -> 2-D Lookup Table6/1
  Product5/1 -> Add7/1
  2-D Lookup Table7/1 -> Product2/1
  Data Type Conversion1/1 -> Add4/2, Add6/2, Add5/2, Add3/2, Add2/2
  [breakpoint2] -> 2-D Lookup Table8/2
  Product/1 -> Product5/2
  Subsystem5/1(Out1) -> Product4/2
  [breakpoint2] -> 2-D Lookup Table7/2
  Subsystem2/1(Out1) -> Product1/2
  Constant8/1 -> Add5/1
  Product8/1 -> Add7/4
  Constant7/1 -> Add4/1
  Add4/1 -> Subsystem3/1(In1)
  Subsystem3/1(Out1) -> Product2/2
  Subsystem4/1(Out1) -> Product3/2
  Product1/1 -> Product6/2
  Add2/1 -> Subsystem1/1(In1)
  [breakpoint1] -> 2-D Lookup Table8/1
  [breakpoint2] -> 2-D Lookup Table6/2
  2-D Lookup Table5/1 -> Product/1
  Constant5/1 -> Add2/1
  2-D Lookup Table8/1 -> Product3/1
  Constant6/1 -> Add3/1
  Add6/1 -> Subsystem5/1(In1)
  Add5/1 -> Subsystem4/1(In1)
  Product3/1 -> Product8/2
  [breakpoint2] -> 2-D Lookup Table9/2
  Add3/1 -> Subsystem2/1(In1)
  Add7/1 -> Data Type Conversion/1
  2-D Lookup Table6/1 -> Product1/1
  Product7/1 -> Add7/3
  2-D Lookup Table9/1 -> Product4/1
  Product6/1 -> Add7/2
  breakpoint1/1 -> [breakpoint1]
  breakpoint2/1 -> [breakpoint2]
  XCP/1(Out1) -> Data Type Conversion1/1
  Constant/1 -> Product5/1
  Constant1/1 -> Product6/1
  Constant2/1 -> Product7/1
  Constant3/1 -> Product8/1
  Constant4/1 -> Product9/1
  md_u8Blw/1 -> XCP/1(md_u8Blw)
  Data Type Conversion/1 -> Flow2Rpm/1

== system ScriptDemo/Create/createMerge/After/SM3SM23/ID26263_SM3Error/SM3HPErr/CalEvapReqOffset ==
  note: 偏差限制在0~9°内
  note: SM3EvapReqOffset每1s增加
  note: 需要对蒸发器请求温度补偿
  note: 不需要对蒸发器请求温度补偿
  note: 偏差限制在0~9°内
  note: TODO: 端口1一直无法false
  sTmSigProces_Te_s32EvapFanReqRamp : Inport  OutDataTypeStr=single
  xTmComprCtrl_B_ModeChanged : Inport  Port=2  OutDataTypeStr=boolean
  rTmComprCtrl_Te_s32SM3BattError : Inport  Port=3  OutDataTypeStr=single
  xTmComprCtrl_B_SM3ErrNeedOffset : Inport  Port=4  OutDataTypeStr=boolean
  Add2 : Sum  Inputs=+-  SaturateOnIntegerOverflow=on
  Add4 : Sum
  Add6 : Sum  Inputs=+-  SaturateOnIntegerOverflow=on
  Constant : Constant  Value=0  OutDataTypeStr=single
  Constant10 : Constant  Value=cTmComprCtrl_Te_i16SM3BatDiffStartEvapDecOffset
  Constant11 : Constant  Value=cTmComprCtrl_Te_s32SM3EvapDecOffsetStep
  Constant12 : Constant  Value=cTmSwArch_t_s32SampleTime
  Constant14 : Constant  Value=cTmComprCtrl_Te_i16SM3EvapLo
  Constant7 : Constant  Value=0
  Constant8 : Constant  Value=cTmComprCtrl_Te_s32SM3EvapOffsetResetStep
  Constant9 : Constant  Value=cTmSwArch_t_s32SampleTime
  Logical Operator1 : Logic  AllPortsSameDT=off  OutDataTypeStr=boolean
  Product : Product
  Product1 : Product
  Relational Operator5 : RelationalOperator  Operator=>  OutDataTypeStr=boolean  RndMeth=Simplest  InputSameDT=off
  Relational Operator7 : RelationalOperator  OutDataTypeStr=boolean  RndMeth=Simplest  InputSameDT=off
  Switch : Switch  Criteria=u2 ~= 0  SaturateOnIntegerOverflow=off  InputSameDT=off
  Switch2 : Switch  Criteria=u2 ~= 0  SaturateOnIntegerOverflow=off  InputSameDT=off
  Switch3 : Switch  Criteria=u2 > Threshold  SaturateOnIntegerOverflow=off  InputSameDT=off
  Switch4 : Switch  Criteria=u2 ~= 0  SaturateOnIntegerOverflow=off  InputSameDT=off
  Unit Delay2 : UnitDelay  SampleTime=-1  HasFrameUpgradeWarning=on
  rTmComprCtrl_Te_s32SM3EvapReqOffset : Outport
  wires:
  Constant11/1 -> Product1/1
  Constant8/1 -> Product/1
  Add4/1 -> Switch4/1
  Unit Delay2/1 -> [rTmComprCtrl_Te_s32SM3EvapReqOffset]
  Product1/1 -> Add4/2
  Constant7/1 -> Switch3/3
  Relational Operator5/1 -> Logical Operator1/1
  [rTmComprCtrl_Te_s32SM3EvapReqOffset] -> Switch3/2
  Constant9/1 -> Product/2
  Switch/1 -> rTmComprCtrl_Te_s32SM3EvapReqOffset/1, Unit Delay2/1  "rTmComprCtrl_Te_s32SM3EvapReqOffset"
  Add2/1 -> Switch3/1
  Constant10/1 -> Relational Operator5/2
  [rTmComprCtrl_Te_s32SM3EvapReqOffset] -> Add4/1
  Constant12/1 -> Product1/2
  [sTmSigProces_Te_s32EvapFanReqRamp] -> Add6/1
  Relational Operator7/1 -> Logical Operator1/2
  Logical Operator1/1 -> Switch4/2
  Product/1 -> Add2/2
  [rTmComprCtrl_Te_s32SM3EvapReqOffset] -> Switch4/3
  [rTmComprCtrl_Te_s32SM3EvapReqOffset] -> Add6/2
  Add6/1 -> Relational Operator7/1
  Constant14/1 -> Relational Operator7/2
  Switch3/1 -> Switch2/3
  [rTmComprCtrl_Te_s32SM3EvapReqOffset] -> Add2/1
  Switch4/1 -> Switch2/1
  sTmSigProces_Te_s32EvapFanReqRamp/1 -> [sTmSigProces_Te_s32EvapFanReqRamp]
  [xTmComprCtrl_B_ModeChanged] -> Switch/2
  Constant/1 -> Switch/1
  Switch2/1 -> Switch/3
  xTmComprCtrl_B_ModeChanged/1 -> [xTmComprCtrl_B_ModeChanged]
  [xTmComprCtrl_B_SM3ErrNeedOffset] -> Switch2/2
  [rTmComprCtrl_Te_s32SM3BattError] -> Relational Operator5/1
  rTmComprCtrl_Te_s32SM3BattError/1 -> [rTmComprCtrl_Te_s32SM3BattError]
  xTmComprCtrl_B_SM3ErrNeedOffset/1 -> [xTmComprCtrl_B_SM3ErrNeedOffset]

== system ScriptDemo/Create/createMerge/After/SM3SM23/ID26263_SM3Error/SM3HPErr/NegAndPosCheck 1 ==
  SetPoint : Inport
  Acture : Inport  Port=2
  Compare To Constant : simulink/Logic and Bit Operations/Compare To Constant  relop=>=  const=0  OutDataTypeStr=boolean
  Data Type Conversion : DataTypeConversion  SaturateOnIntegerOverflow=off  RndMeth=Floor
  Data Type Conversion1 : DataTypeConversion  SaturateOnIntegerOverflow=off  RndMeth=Floor
  Data Type Conversion2 : DataTypeConversion  SaturateOnIntegerOverflow=off  RndMeth=Floor
  Sum : Sum  Inputs=|-+  OutDataTypeStr=Inherit: Same as first input
  Dvt : Outport  VectorParamsAs1DForOutWhenUnconnected=off
  Dvt_PosFlag : Outport  Port=2  VectorParamsAs1DForOutWhenUnconnected=off
  wires:
  Data Type Conversion2/1 -> Dvt/1, Compare To Constant/1
  Data Type Conversion1/1 -> Sum/2
  Data Type Conversion/1 -> Sum/1
  Compare To Constant/1 -> Dvt_PosFlag/1
  Sum/1 -> Data Type Conversion2/1
  Acture/1 -> Data Type Conversion1/1
  SetPoint/1 -> Data Type Conversion/1

== system ScriptDemo/Create/createMerge/After/SM3SM23/ID26263_SM3Error/SM3HPErr/isNeedOffset ==
  sTmSigProces_Te_s32EvapFanFilter : Inport  OutDataTypeStr=single
  sTmIn_Te_s32HvBattCooltTReq : Inport  Port=2  OutDataTypeStr=single
  sTmSigProces_Te_s32HvBattCooltTFilter : Inport  Port=3  OutDataTypeStr=single
  Add3 : Sum  Inputs=+-
  Constant1 : Constant  Value=cTmComprCtrl_Te_s32SM3TimeForEntEvapDecOffset
  Constant2 : Constant  Value=cTmComprCtrl_Te_i16SM3EvapLo
  Logical Operator : Logic  AllPortsSameDT=off  OutDataTypeStr=boolean
  Logical Operator2 : Logic  Operator=NOT  AllPortsSameDT=off  OutDataTypeStr=boolean
  Relational Operator3 : RelationalOperator  Operator=>  OutDataTypeStr=boolean  RndMeth=Simplest  InputSameDT=off
  Relay : Relay  OnSwitchValue=cTmComprCtrl_Te_i16SM3TBatDiffEntEvapDecOffset  OffSwitchValue=cTmComprCtrl_Te_i16SM3TBatDiffEntEvapDecOffsetQuit
  Terminator3 : Terminator
  Timer Running2 : Subsystem  AncestorBlock=UXFD_Lib/CCM/Timer Running  mask(Timer Running NGCC v1.0){timeDataType=uint16, RunnablePeriod=No_Runnable_Period}
      mask prompts: timeDataType "Time data type:"; RunnablePeriod "SWC Sampling Time Parameter:"
      mask help:
      | If Start (1) is true, the timer is started.
      | The timer works as a "set/reset"-functionality, i.e. start does not have to be "true" continuously to keep the timer running.
      | Timer will be reset to 0 if Reset (2) is true.
      | TimerFinished (output) specifies if the timer is finished (boolean).
      | If Time (3) is set to zero, this block will function as a set-reset latch.
      | Reset is always master over Start.
      |
      | TmrRunng (output 2) will be set when timer is activated.
      |
      | Mx-VDev tested: Yes
      mask init:
      | %Set sample time
      | blkName = gcb;
      | modelName = char(regexp(blkName,'(\w*)_(?:Runnable|lib)','tokens','once'));
      | if isempty(modelName)
      |     modelName = 'No';
      | end
      | timeParameter = [modelName '_Runnable_Period'];
      | set_param(blkName, 'RunnablePeriod',timeParameter);
      mask TypeOptions timeDataType: uint8 | uint16 | uint32 | single
      mask Display:
      | try
      |     image(imread([CCMConfig.GetRootDir '\Shared\SimulinkLibrary\Images\timer.bmp']))
      | catch
      |     fprintf('Timer\nHoldable')
      | end
      | port_label('output',1,'TmrFinshd')
      | port_label('output',2,'TmrRunng')
      | port_label('input',1,'Start')
      | port_label('input',2,'Reset')
      | port_label('input',3,'Time')
  xTmComprCtrl_B_SM3ErrNeedOffset : Outport  OutDataTypeStr=boolean
  rTmComprCtrl_Te_s32SM3BattError : Outport  Port=2  OutDataTypeStr=single
  wires:
  Constant1/1 -> Timer Running2/3(Time)
  Logical Operator/1 -> Timer Running2/1(Start), Logical Operator2/1
  Timer Running2/1(TimerFinished) -> [xTmComprCtrl_B_SM3ErrNeedOffset]
  [sTmSigProces_Te_s32EvapFanFilter] -> Relational Operator3/1
  Constant2/1 -> Relational Operator3/2
  Timer Running2/2(TimerRunning) -> Terminator3/1
  Logical Operator2/1 -> Timer Running2/2(Reset)
  [xTmComprCtrl_B_SM3ErrNeedOffset] -> xTmComprCtrl_B_SM3ErrNeedOffset/1  "xTmComprCtrl_B_SM3ErrNeedOffset"
  [rTmComprCtrl_Te_s32SM3BattError] -> Relay/1
  Relay/1 -> Logical Operator/1
  Relational Operator3/1 -> Logical Operator/2
  sTmSigProces_Te_s32EvapFanFilter/1 -> [sTmSigProces_Te_s32EvapFanFilter]
  Add3/1 -> [rTmComprCtrl_Te_s32SM3BattError]  "rTmComprCtrl_Te_s32SM3BattError"
  [sTmSigProces_Te_s32HvBattCooltTFilter] -> Add3/1
  [sTmIn_Te_s32HvBattCooltTReq] -> Add3/2
  sTmIn_Te_s32HvBattCooltTReq/1 -> [sTmIn_Te_s32HvBattCooltTReq]
  sTmSigProces_Te_s32HvBattCooltTFilter/1 -> [sTmSigProces_Te_s32HvBattCooltTFilter]
  [rTmComprCtrl_Te_s32SM3BattError] -> rTmComprCtrl_Te_s32SM3BattError/1  "rTmComprCtrl_Te_s32SM3BattError"

== system ScriptDemo/Create/createMerge/After/SM3SM23/ID26263_SM3Error/SM3NHPErr/NegAndPosCheck 2 ==
  SetPoint : Inport
  Acture : Inport  Port=2
  Compare To Constant : simulink/Logic and Bit Operations/Compare To Constant  relop=>=  const=0  OutDataTypeStr=boolean
  Data Type Conversion : DataTypeConversion  SaturateOnIntegerOverflow=off  RndMeth=Floor
  Data Type Conversion1 : DataTypeConversion  SaturateOnIntegerOverflow=off  RndMeth=Floor
  Data Type Conversion2 : DataTypeConversion  SaturateOnIntegerOverflow=off  RndMeth=Floor
  Sum : Sum  Inputs=|-+  OutDataTypeStr=Inherit: Same as first input
  Dvt : Outport  VectorParamsAs1DForOutWhenUnconnected=off
  Dvt_PosFlag : Outport  Port=2  VectorParamsAs1DForOutWhenUnconnected=off
  wires:
  Data Type Conversion2/1 -> Dvt/1, Compare To Constant/1
  Data Type Conversion1/1 -> Sum/2
  Data Type Conversion/1 -> Sum/1
  Compare To Constant/1 -> Dvt_PosFlag/1
  Sum/1 -> Data Type Conversion2/1
  Acture/1 -> Data Type Conversion1/1
  SetPoint/1 -> Data Type Conversion/1

== system ScriptDemo/Create/createMerge/After/SM3SM23/ID26263_SM3Error/SM3NHPErr/NegAndPosCheck 3 ==
  SetPoint : Inport
  Acture : Inport  Port=2
  Compare To Constant : simulink/Logic and Bit Operations/Compare To Constant  relop=>=  const=0  OutDataTypeStr=boolean
  Data Type Conversion : DataTypeConversion  SaturateOnIntegerOverflow=off  RndMeth=Floor
  Data Type Conversion1 : DataTypeConversion  SaturateOnIntegerOverflow=off  RndMeth=Floor
  Data Type Conversion2 : DataTypeConversion  SaturateOnIntegerOverflow=off  RndMeth=Floor
  Sum : Sum  Inputs=|-+  OutDataTypeStr=Inherit: Same as first input
  Dvt : Outport  VectorParamsAs1DForOutWhenUnconnected=off
  Dvt_PosFlag : Outport  Port=2  VectorParamsAs1DForOutWhenUnconnected=off
  wires:
  Data Type Conversion2/1 -> Dvt/1, Compare To Constant/1
  Data Type Conversion1/1 -> Sum/2
  Data Type Conversion/1 -> Sum/1
  Compare To Constant/1 -> Dvt_PosFlag/1
  Sum/1 -> Data Type Conversion2/1
  Acture/1 -> Data Type Conversion1/1
  SetPoint/1 -> Data Type Conversion/1

== system ScriptDemo/Create/createMerge/After/SM3SM23/SM3_Ki/SM1Ki/tableChoose ==
  note: 快充
  note: 非快充，超充
  note: 电池有主动制冷需求
  note: 电池非正常制冷
  note: 超充
  note: 电池有主动制冷需求
  sTmSigProces_D_u8BattThermReq : Inport
  sTmIn_D_u8DCChrgSt : Inport  Port=2
  tab1 : Inport  Port=3
  tab2 : Inport  Port=4
  tab3 : Inport  Port=5
  Compare To Constant : simulink/Logic and Bit Operations/Compare To Constant  relop===  const=2  OutDataTypeStr=boolean
  Compare To Constant1 : simulink/Logic and Bit Operations/Compare To Constant  relop===  const=12  OutDataTypeStr=boolean
  Compare To Constant2 : simulink/Logic and Bit Operations/Compare To Constant  relop===  const=5  OutDataTypeStr=boolean
  Switch2 : Switch  Criteria=u2 ~= 0  SaturateOnIntegerOverflow=off  InputSameDT=off
  Switch4 : Switch  Criteria=u2 ~= 0  SaturateOnIntegerOverflow=off  InputSameDT=off
  Switch5 : Switch  Criteria=u2 ~= 0  SaturateOnIntegerOverflow=off  InputSameDT=off
  电池无主动制冷需求 : Constant  Value=0  OutDataTypeStr=uint16
  out : Outport  OutDataTypeStr=uint16
  wires:
  Compare To Constant1/1 -> Switch5/2
  tab1/1 -> Switch5/3
  tab3/1 -> Switch5/1
  tab2/1 -> Switch4/1
  sTmIn_D_u8DCChrgSt/1 -> Compare To Constant/1, Compare To Constant1/1
  Switch5/1 -> Switch4/3
  sTmSigProces_D_u8BattThermReq/1 -> Compare To Constant2/1
  Compare To Constant2/1 -> Switch2/2
  电池无主动制冷需求/1 -> Switch2/3
  Switch2/1 -> out/1
  Switch4/1 -> Switch2/1
  Compare To Constant/1 -> Switch4/2
